simulink model "AED2D"  (R2018b)
settings: Solver=FixedStepAuto  StartTime=0.0  StopTime=Tfim  FixedStep=0.001  MaxStep=0.001  RelTol=1e-3
values from neighbouring files (symbols this model uses):
  D = DadosCGInercia(D)    [PlotGMax.m]    (also in S.mat = ; VooUnico.m; VooUnico6DOF.m)
  dados =     [S.mat]
  g = 9.8    [plot_exocet_6dof.m]
  M_CD = [8.341 8.24 8.141 8.043 7.946 7.851 7.76 7.674 7.595 7.523 7.46 7.4 ... (1365 elements, 21x5x13)]    [S.mat]
  M_CM = [42.757 43.119 43.498 43.905 44.357 44.839 45.319 45.775 46.191 46.536 46.769 46.963 ... (1365 elements, 21x5x13)]    [S.mat]
  M_CMQ = [-1543.746 -1552.906 -1559.915 -1565.64 -1570.662 -1573.443 -1572.931 -1569.859 -1564.198 -1553.449 -1535.22 -1514.504 ... (1365 elements, 21x5x13)]    [S.mat]
  M_CN = [-21.126 -21.088 -21.046 -20.997 -20.94 -20.877 -20.812 -20.749 -20.692 -20.644 -20.613 -20.587 ... (1365 elements, 21x5x13)]    [S.mat]
  R2D = 57.2957795131    [S.mat]    (also in VooUnico.m; VooUnico6DOF.m; plot6DOF.m; plot_exocet_6dof.m)
undefined symbols (not defined in the file or in its folder): AclnMax, AltCruz, anp, dist_manobra, Dlt_max, Dlt_max_roll, F_propB, F_propS, GanhoAtit, M_CMAD, M_CNAD, M_CNQ, manobra, Newton, ng, p0, phi0, psi0, psimaxAD, q0, r0, RampaMax, Raphson, sat_integAP, sigmaYmaxAD, sigmaZmaxAD, T_acel_k_ext, T_acel_k_int, T_at_k_ext, T_at_k_int, theta0, thetamaxAD, TLaser, Tresp, TTrav, vet_altitude, vet_Mach, vet_x_CG, Vxa0, Vya0, Vza0, Xa0, Ya0, Za0
libraries: simulink x11, sharedutil x4, aerolibasang x4, vrlib x3, shared6dof x2, aerolibatmos2 x1, dspmtrx3 x1
(part 2 of 2)

== system AED2D/Dinâmica 6DOF/Aerodinâmica/Subsystem ==
  dltz : Inport
  "Mach " : Inport  Port=2
  alfa : Inport  Port=3
  qS : Inport  Port=4
  q : Inport  Port=5
  d2V : Inport  Port=6
  alfap : Inport  Port=7
  Add : Sum  Inputs=+++
  Gain1 : Gain  Gain=R2D
  Gain2 : Gain  Gain=R2D
  Gain3 : Gain  Gain=-1
  Product2 : Product
  Product4 : Product  Inputs=3
  Product5 : Product  Inputs=3
  n-D Lookup Table : Lookup_n-D  NumberOfTableDimensions=3  BreakpointsForDimension1=dados.delta  BreakpointsForDimension2=dados.mach  BreakpointsForDimension3=dados.alpha  Table=M_CN  ExtrapMethod=Clip  InternalRulePriority=Speed  RndMeth=Simplest  InputSameDT=on
  n-D Lookup Table1 : Lookup_n-D  NumberOfTableDimensions=3  BreakpointsForDimension1=dados.delta  BreakpointsForDimension2=dados.mach  BreakpointsForDimension3=dados.alpha  Table=M_CNQ  ExtrapMethod=Clip  InternalRulePriority=Speed  RndMeth=Simplest  InputSameDT=on
  n-D Lookup Table2 : Lookup_n-D  NumberOfTableDimensions=3  BreakpointsForDimension1=dados.delta  BreakpointsForDimension2=dados.mach  BreakpointsForDimension3=dados.alpha  Table=M_CNAD  ExtrapMethod=Clip  InternalRulePriority=Speed  RndMeth=Simplest  InputSameDT=on
  Fz : Outport
  wires:
  n-D Lookup Table1/1 -> Product4/1
  d2V/1 -> Product5/3, Product4/3
  n-D Lookup Table2/1 -> Product5/1
  q/1 -> Product4/2
  alfap/1 -> Product5/2
  "Mach "/1 -> n-D Lookup Table/2, n-D Lookup Table2/2, n-D Lookup Table1/2
  dltz/1 -> Gain2/1
  alfa/1 -> Gain1/1
  Product5/1 -> Add/3
  Product4/1 -> Add/2
  Product2/1 -> Gain3/1
  Add/1 -> Product2/1
  qS/1 -> Product2/2
  Gain2/1 -> n-D Lookup Table2/1, n-D Lookup Table1/1, n-D Lookup Table/1
  Gain1/1 -> n-D Lookup Table2/3, n-D Lookup Table1/3, n-D Lookup Table/3
  n-D Lookup Table/1 -> Add/1
  Gain3/1 -> Fz/1

== system AED2D/Dinâmica 6DOF/Aerodinâmica/Subsystem1 ==
  "dlty " : Inport
  Mach : Inport  Port=2
  beta : Inport  Port=3
  qS : Inport  Port=4
  d2V : Inport  Port=5
  r : Inport  Port=6
  betap : Inport  Port=7
  Add : Sum  Inputs=+++
  Gain2 : Gain  Gain=-R2D
  Gain3 : Gain  Gain=R2D
  Product1 : Product
  Product2 : Product  Inputs=3
  Product5 : Product  Inputs=3
  n-D Lookup Table : Lookup_n-D  NumberOfTableDimensions=3  BreakpointsForDimension1=dados.delta  BreakpointsForDimension2=dados.mach  BreakpointsForDimension3=dados.alpha  Table=M_CN  ExtrapMethod=Clip  InternalRulePriority=Speed  RndMeth=Simplest  InputSameDT=on
  n-D Lookup Table1 : Lookup_n-D  NumberOfTableDimensions=3  BreakpointsForDimension1=dados.delta  BreakpointsForDimension2=dados.mach  BreakpointsForDimension3=dados.alpha  Table=M_CNAD  ExtrapMethod=Clip  InternalRulePriority=Speed  RndMeth=Simplest  InputSameDT=on
  n-D Lookup Table2 : Lookup_n-D  NumberOfTableDimensions=3  BreakpointsForDimension1=dados.delta  BreakpointsForDimension2=dados.mach  BreakpointsForDimension3=dados.alpha  Table=M_CNAD  ExtrapMethod=Clip  InternalRulePriority=Speed  RndMeth=Simplest  InputSameDT=on
  Fy : Outport
  wires:
  Add/1 -> Product1/1
  beta/1 -> Gain2/1
  "dlty "/1 -> Gain3/1
  Mach/1 -> n-D Lookup Table2/2, n-D Lookup Table1/2, n-D Lookup Table/2
  Product5/1 -> Add/2
  qS/1 -> Product1/2
  Gain3/1 -> n-D Lookup Table2/1, n-D Lookup Table1/1, n-D Lookup Table/1
  n-D Lookup Table/1 -> Add/1
  d2V/1 -> Product2/3, Product5/2
  n-D Lookup Table1/1 -> Product5/1
  Gain2/1 -> n-D Lookup Table2/3, n-D Lookup Table1/3, n-D Lookup Table/3
  r/1 -> Product5/3
  Product1/1 -> Fy/1
  Product2/1 -> Add/3
  n-D Lookup Table2/1 -> Product2/1
  betap/1 -> Product2/2

== system AED2D/Dinâmica 6DOF/Aerodinâmica/Subsystem2 ==
  alfa : Inport
  beta : Inport  Port=2
  qS : Inport  Port=3
  dlty : Inport  Port=4
  dltz : Inport  Port=5
  "Mach " : Inport  Port=6
  Add : Sum  Inputs=++-
  Constant : Constant  Value=0
  Gain : Gain  Gain=-1
  Gain{1..4} (4 alike) : Gain  Gain=R2D
  Product : Product
  n-D Lookup Table : Lookup_n-D  NumberOfTableDimensions=3  BreakpointsForDimension1=dados.delta  BreakpointsForDimension2=dados.mach  BreakpointsForDimension3=dados.alpha  Table=M_CD  ExtrapMethod=Clip  InternalRulePriority=Speed  RndMeth=Simplest  InputSameDT=on
  n-D Lookup Table1 : Lookup_n-D  NumberOfTableDimensions=3  BreakpointsForDimension1=dados.delta  BreakpointsForDimension2=dados.mach  BreakpointsForDimension3=dados.alpha  Table=M_CD  ExtrapMethod=Clip  InternalRulePriority=Speed  RndMeth=Simplest  InputSameDT=on
  n-D Lookup Table2 : Lookup_n-D  NumberOfTableDimensions=3  BreakpointsForDimension1=dados.delta  BreakpointsForDimension2=dados.mach  BreakpointsForDimension3=dados.alpha  Table=M_CD  ExtrapMethod=Clip  InternalRulePriority=Speed  RndMeth=Simplest  InputSameDT=on
  Fx : Outport
  wires:
  "Mach "/1 -> n-D Lookup Table2/2, n-D Lookup Table1/2, n-D Lookup Table/2
  dltz/1 -> Gain3/1
  alfa/1 -> Gain2/1
  dlty/1 -> Gain4/1
  beta/1 -> Gain1/1
  n-D Lookup Table/1 -> Add/1
  n-D Lookup Table1/1 -> Add/2
  Add/1 -> Gain/1
  qS/1 -> Product/2
  Gain3/1 -> n-D Lookup Table/1
  Gain2/1 -> n-D Lookup Table/3
  Gain4/1 -> n-D Lookup Table1/1
  Gain1/1 -> n-D Lookup Table1/3
  Constant/1 -> n-D Lookup Table2/3, n-D Lookup Table2/1
  Gain/1 -> Product/1
  n-D Lookup Table2/1 -> Add/3
  Product/1 -> Fx/1

== system AED2D/Dinâmica 6DOF/Aerodinâmica/Subsystem3 ==
  dlty : Inport
  Mach : Inport  Port=2
  beta : Inport  Port=3
  qSd : Inport  Port=4
  r : Inport  Port=5
  d2V : Inport  Port=6
  betap : Inport  Port=7
  Add : Sum  Inputs=+++
  Gain1 : Gain  Gain=-R2D
  Gain2 : Gain  Gain=R2D
  Product1 : Product  Inputs=3
  Product4 : Product  Inputs=3
  Product6 : Product
  n-D Lookup Table : Lookup_n-D  NumberOfTableDimensions=3  BreakpointsForDimension1=dados.delta  BreakpointsForDimension2=dados.mach  BreakpointsForDimension3=dados.alpha  Table=M_CM  ExtrapMethod=Clip  InternalRulePriority=Speed  RndMeth=Simplest  InputSameDT=on
  n-D Lookup Table1 : Lookup_n-D  NumberOfTableDimensions=3  BreakpointsForDimension1=dados.delta  BreakpointsForDimension2=dados.mach  BreakpointsForDimension3=dados.alpha  Table=M_CMQ  ExtrapMethod=Clip  InternalRulePriority=Speed  RndMeth=Simplest  InputSameDT=on
  n-D Lookup Table2 : Lookup_n-D  NumberOfTableDimensions=3  BreakpointsForDimension1=dados.delta  BreakpointsForDimension2=dados.mach  BreakpointsForDimension3=dados.alpha  Table=M_CMAD  ExtrapMethod=Clip  InternalRulePriority=Speed  RndMeth=Simplest  InputSameDT=on
  N : Outport
  wires:
  d2V/1 -> Product1/2, Product4/3
  Product6/1 -> N/1
  Add/1 -> Product6/1
  qSd/1 -> Product6/2
  r/1 -> Product4/2
  dlty/1 -> Gain2/1
  Mach/1 -> n-D Lookup Table2/2, n-D Lookup Table1/2, n-D Lookup Table/2
  beta/1 -> Gain1/1
  Product4/1 -> Add/2
  Gain2/1 -> n-D Lookup Table1/1, n-D Lookup Table2/1, n-D Lookup Table/1
  Gain1/1 -> n-D Lookup Table2/3, n-D Lookup Table1/3, n-D Lookup Table/3
  n-D Lookup Table/1 -> Add/1
  n-D Lookup Table1/1 -> Product4/1
  n-D Lookup Table2/1 -> Product1/1
  betap/1 -> Product1/3
  Product1/1 -> Add/3

== system AED2D/Dinâmica 6DOF/Aerodinâmica/Subsystem4 ==
  dltz : Inport
  Mach : Inport  Port=2
  alfa : Inport  Port=3
  qSd : Inport  Port=4
  q : Inport  Port=5
  d2V : Inport  Port=6
  alfap : Inport  Port=7
  Add : Sum  Inputs=+++
  Gain1 : Gain  Gain=R2D
  Gain2 : Gain  Gain=R2D
  Product4 : Product  Inputs=3
  Product5 : Product  Inputs=3
  Product6 : Product
  n-D Lookup Table : Lookup_n-D  NumberOfTableDimensions=3  BreakpointsForDimension1=dados.delta  BreakpointsForDimension2=dados.mach  BreakpointsForDimension3=dados.alpha  Table=M_CM  ExtrapMethod=Clip  InternalRulePriority=Speed  RndMeth=Simplest  InputSameDT=on
  n-D Lookup Table1 : Lookup_n-D  NumberOfTableDimensions=3  BreakpointsForDimension1=dados.delta  BreakpointsForDimension2=dados.mach  BreakpointsForDimension3=dados.alpha  Table=M_CMQ  ExtrapMethod=Clip  InternalRulePriority=Speed  RndMeth=Simplest  InputSameDT=on
  n-D Lookup Table2 : Lookup_n-D  NumberOfTableDimensions=3  BreakpointsForDimension1=dados.delta  BreakpointsForDimension2=dados.mach  BreakpointsForDimension3=dados.alpha  Table=M_CMAD  ExtrapMethod=Clip  InternalRulePriority=Speed  RndMeth=Simplest  InputSameDT=on
  M : Outport
  wires:
  d2V/1 -> Product4/3, Product5/3
  Product6/1 -> M/1
  Add/1 -> Product6/1
  qSd/1 -> Product6/2
  q/1 -> Product4/2
  alfap/1 -> Product5/2
  dltz/1 -> Gain2/1
  alfa/1 -> Gain1/1
  Product4/1 -> Add/2
  Product5/1 -> Add/3
  Gain2/1 -> n-D Lookup Table2/1, n-D Lookup Table1/1, n-D Lookup Table/1
  Gain1/1 -> n-D Lookup Table2/3, n-D Lookup Table1/3, n-D Lookup Table/3
  n-D Lookup Table/1 -> Add/1
  n-D Lookup Table1/1 -> Product4/1
  n-D Lookup Table2/1 -> Product5/1
  Mach/1 -> n-D Lookup Table2/2, n-D Lookup Table1/2, n-D Lookup Table/2

== system AED2D/Dinâmica 6DOF/Aerodinâmica/Subsystem6 ==
  Forces : Inport
  CRM : Inport  Port=2
  CG : Inport  Port=3
  Moments CRM : Inport  Port=4
  3x3 Cross Product : sharedutil/3x3 Cross Product
      settings: SourceProductBaseCode=AE
  Sum : Sum  Inputs=|+-  SaturateOnIntegerOverflow=on
  Sum1 : Sum  Inputs=|++  SaturateOnIntegerOverflow=on
  To Workspace : ToWorkspace  VariableName=Delta  SaveFormat=Timeseries  SampleTime=-1
  Moments CG : Outport
  wires:
  CRM/1 -> Sum/1
  CG/1 -> Sum/2
  Sum/1 -> 3x3 Cross Product/1, To Workspace/1
  Forces/1 -> 3x3 Cross Product/2
  Moments CRM/1 -> Sum1/2
  Sum1/1 -> Moments CG/1
  3x3 Cross Product/1 -> Sum1/1

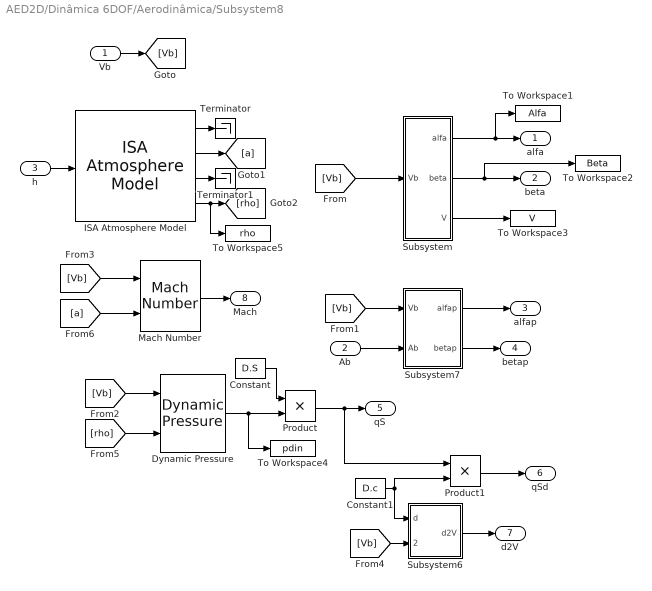
== system AED2D/Dinâmica 6DOF/Aerodinâmica/Subsystem8 ==
  Vb : Inport
  Ab : Inport  Port=2
  h : Inport  Port=3
  Constant : Constant  Value=D.S
  Constant1 : Constant  Value=D.c
  Dynamic Pressure : aerolibasang/Dynamic Pressure
  ISA Atmosphere Model : aerolibatmos2/ISA Atmosphere Model  custom=off  g=9.80665  gamma=1.4  R=287.0531  L=0.0065  h_trop=11000  h_strat=20000  rho0=1.225  P0=101325  T0=288.15  h0=0
      settings: SourceProductName=Aerospace Blockset
  Mach Number : aerolibasang/Mach Number
      settings: SourceProductName=Aerospace Blockset  SourceProductBaseCode=AE
  Product : Product
  Product1 : Product
  Subsystem : Subsystem
  Subsystem6 : Subsystem
  Subsystem7 : Subsystem
  Terminator : Terminator
  Terminator1 : Terminator
  To Workspace1 : ToWorkspace  VariableName=Alfa  SaveFormat=Timeseries  SampleTime=-1
  To Workspace2 : ToWorkspace  VariableName=Beta  SaveFormat=Timeseries  SampleTime=-1
  To Workspace3 : ToWorkspace  VariableName=V  SaveFormat=Timeseries  SampleTime=-1
  To Workspace4 : ToWorkspace  VariableName=pdin  SaveFormat=Timeseries  SampleTime=-1
  To Workspace5 : ToWorkspace  VariableName=rho  SaveFormat=Timeseries  SampleTime=-1
  alfa : Outport
  beta : Outport  Port=2
  alfap : Outport  Port=3
  betap : Outport  Port=4
  qS : Outport  Port=5
  qSd : Outport  Port=6
  d2V : Outport  Port=7
  Mach : Outport  Port=8
  wires:
  Subsystem7/2(betap) -> betap/1
  Subsystem7/1(alfap) -> alfap/1
  h/1 -> ISA Atmosphere Model/1
  Constant/1 -> Product/1
  Dynamic Pressure/1 -> To Workspace4/1, Product/2
  ISA Atmosphere Model/4 -> To Workspace5/1, [rho]
  Constant1/1 -> Product1/2, Subsystem6/1(d)
  Product1/1 -> qSd/1
  Subsystem6/1(d2V) -> d2V/1
  Product/1 -> Product1/1, qS/1
  Subsystem/3(V) -> To Workspace3/1
  Subsystem/1(alfa) -> To Workspace1/1, alfa/1
  Subsystem/2(beta) -> beta/1, To Workspace2/1
  Mach Number/1 -> Mach/1
  Vb/1 -> [Vb]
  [Vb] -> Subsystem/1(Vb)
  [Vb] -> Subsystem7/1(Vb)
  [Vb] -> Dynamic Pressure/1
  [Vb] -> Mach Number/1
  [Vb] -> Subsystem6/2(Velocity)
  [rho] -> Dynamic Pressure/2
  [a] -> Mach Number/2
  ISA Atmosphere Model/2 -> [a]
  ISA Atmosphere Model/1 -> Terminator/1
  ISA Atmosphere Model/3 -> Terminator1/1
  Ab/1 -> Subsystem7/2(Ab)

== system AED2D/Guiamento/Navegação Proporcional /Gera Matriz C_CIM ==
  Psi AD : Inport
  Theta AD : Inport  Port=2
  Create 3x3 Matrix : sharedutil/Create 3x3 Matrix
  Fc22 : Fcn  Expr=u(2)
  Fcn11 : Fcn  Expr=u(4)*u(2)
  Fcn12 : Fcn  Expr=u(1)*u(4)
  Fcn13 : Fcn  Expr=-u(3)
  Fcn21 : Fcn  Expr=-u(1)
  Fcn23 : Fcn  Expr=0
  Fcn31 : Fcn  Expr=u(2)*u(3)
  Fcn32 : Fcn  Expr=u(1)*u(3)
  Fcn33 : Fcn  Expr=u(4)
  Mux1 : Mux  Inputs=[1 1 1 1]
  sincos : Trigonometry  Operator=sincos
  sincos1 : Trigonometry  Operator=sincos
  C_CIM : Outport
  wires:
  Fcn33/1 -> Create 3x3 Matrix/9
  Fcn23/1 -> Create 3x3 Matrix/6
  Fc22/1 -> Create 3x3 Matrix/5
  Fcn12/1 -> Create 3x3 Matrix/2
  Fcn21/1 -> Create 3x3 Matrix/4
  Fcn11/1 -> Create 3x3 Matrix/1
  Mux1/1 -> Fcn11/1, Fcn12/1, Fcn13/1, Fcn21/1, Fcn33/1, Fcn32/1, Fcn31/1, Fcn23/1, Fc22/1
  sincos/2 -> Mux1/2
  sincos/1 -> Mux1/1
  Fcn13/1 -> Create 3x3 Matrix/3
  sincos1/2 -> Mux1/4
  Psi AD/1 -> sincos/1
  Theta AD/1 -> sincos1/1
  sincos1/1 -> Mux1/3
  Fcn31/1 -> Create 3x3 Matrix/7
  Fcn32/1 -> Create 3x3 Matrix/8
  Create 3x3 Matrix/1 -> C_CIM/1  "Matriz Rotação C_CIM"

== system AED2D/Guiamento/Navegação Proporcional /Gravidade ==
  DCM : Inport
  Constant1 : Constant  Value=0
  Constant5 : Constant  Value=0
  Constant6 : Constant  Value=-g
  Demux1 : Demux  Outputs=3
  Mux2 : Mux  Inputs=3
  Product1 : Product  Multiplication=Matrix(*)
  Terminator2 : Terminator
  -g_yb1 : Outport
  -g_zb1 : Outport  Port=2
  wires:
  Demux1/2 -> -g_yb1/1
  DCM/1 -> Product1/1
  Constant6/1 -> Mux2/3
  Mux2/1 -> Product1/2
  Constant5/1 -> Mux2/2
  Demux1/1 -> Terminator2/1
  Demux1/3 -> -g_zb1/1
  Constant1/1 -> Mux2/1
  Product1/1 -> Demux1/1

== system AED2D/Dinâmica 6DOF/Aerodinâmica/Subsystem8/Subsystem ==
  Vb : Inport
  Airspeed : Sqrt  AlgorithmType=Newton-Raphson  SaturateOnIntegerOverflow=on
  Demux1 : Demux  Outputs=3
  Incidence : Trigonometry  Operator=atan2
  Incidence1 : Trigonometry  Operator=atan2
  dot : aerolibasang/Incidence, Sideslip, & Airspeed/dot
      settings: SourceProductName=Aerospace Blockset  SourceProductBaseCode=AE
  alfa : Outport
  beta : Outport  Port=2
  V : Outport  Port=3
  wires:
  Demux1/3 -> Incidence/1
  Incidence/1 -> alfa/1
  Vb/1 -> Demux1/1, dot/1
  Demux1/2 -> Incidence1/1
  dot/1 -> Airspeed/1
  Airspeed/1 -> V/1
  Incidence1/1 -> beta/1
  Demux1/1 -> Incidence/2, Incidence1/2

== system AED2D/Dinâmica 6DOF/Aerodinâmica/Subsystem8/Subsystem6 ==
  d : Inport
  Velocity : Inport  Port=2
  Divide : Product  Inputs=*/
  d/(2V) : Gain  Gain=1/2  SaturateOnIntegerOverflow=on  OutDataTypeStr=Inherit: Same as input  ParamDataTypeStr=Inherit: Same as input
  dot : aerolibasang/Dynamic Pressure/dot
      settings: SourceProductName=Aerospace Blockset  SourceProductBaseCode=AE
  vt : Sqrt  AlgorithmType=Newton-Raphson  SaturateOnIntegerOverflow=on
  d2V : Outport  InitialOutput=0
  wires:
  d/(2V)/1 -> d2V/1
  Velocity/1 -> dot/1
  Divide/1 -> d/(2V)/1
  dot/1 -> vt/1
  d/1 -> Divide/1
  vt/1 -> Divide/2

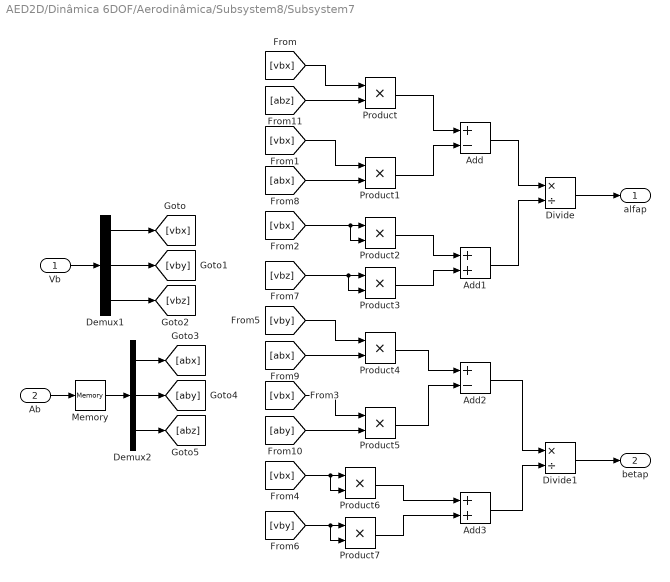
== system AED2D/Dinâmica 6DOF/Aerodinâmica/Subsystem8/Subsystem7 ==
  Vb : Inport
  Ab : Inport  Port=2
  Add : Sum  Inputs=+-
  Add1 : Sum
  Add2 : Sum  Inputs=+-
  Add3 : Sum
  Demux1 : Demux  Outputs=3
  Demux2 : Demux  Outputs=3
  Divide : Product  Inputs=*/
  Divide1 : Product  Inputs=*/
  Memory : Memory
  Product{,1..7} (8 alike) : Product
  alfap : Outport
  betap : Outport  Port=2
  wires:
  Product/1 -> Add/1
  Product1/1 -> Add/2
  Product2/1 -> Add1/1
  Product3/1 -> Add1/2
  Add/1 -> Divide/1
  Add1/1 -> Divide/2
  Divide/1 -> alfap/1
  Product4/1 -> Add2/1
  Divide1/1 -> betap/1
  Product7/1 -> Add3/2
  Add2/1 -> Divide1/1
  Product6/1 -> Add3/1
  Product5/1 -> Add2/2
  Add3/1 -> Divide1/2
  Vb/1 -> Demux1/1
  Demux1/1 -> [vbx]
  Demux1/2 -> [vby]
  Demux1/3 -> [vbz]
  [vbx] -> Product/1
  [vbx] -> Product1/1
  [vbx] -> Product2/2, Product2/1
  [vbx] -> Product5/1
  [vbx] -> Product6/2, Product6/1
  [vby] -> Product4/1
  [vby] -> Product7/2, Product7/1
  [vbz] -> Product3/2, Product3/1
  Memory/1 -> Demux2/1
  Ab/1 -> Memory/1
  Demux2/1 -> [abx]
  Demux2/2 -> [aby]
  Demux2/3 -> [abz]
  [abx] -> Product1/2
  [abx] -> Product4/2
  [aby] -> Product5/2
  [abz] -> Product/2
